simulink model "Model6"  (Simulink 8.1)
settings: Solver=ode15s  StartTime=StartTime  StopTime=StopTime  FixedStep=FixedStepSize  MaxStep=0.01  RelTol=1e-3
undefined symbols (not defined in the file or in its folder): D, dP, Ki, KOnline, Kp, M, R, TCH
settings Model: Creator=posq  LastModifiedBy=mfal  ExtModeAutoUpdateStatusClock=off
settings DataIOCC: SaveTime=off
settings OptimizationCC: ExpressionDepthLimit=128  InitFltsAndDblsToZero=on
settings DebuggingCC: SaveWithParameterizedLinksMsg=none  MultiTaskCondExecSysMsg=none  StrictBusMsg=Warning
settings RTWCC: IncludeERTFirstTime=on

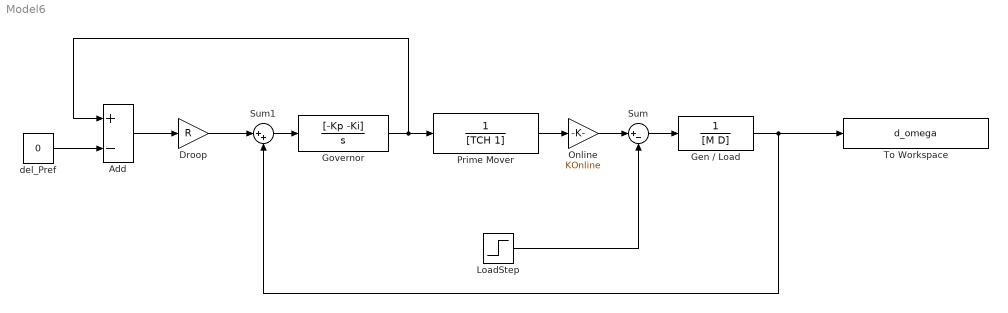
== system Model6 ==
  Add : Sum  Inputs=+-
  Droop : Gain  Gain=R
  Gen / Load : TransferFcn  Denominator=[M D]
  Governor : TransferFcn  Numerator=[-Kp -Ki]  Denominator=[1 0]
  LoadStep : Step  Time=0  After=dP  SampleTime=0
  Online : Gain  Gain=KOnline
  Prime Mover : TransferFcn  Denominator=[TCH 1]
  Sum : Sum  Inputs=|+-
  Sum1 : Sum  Inputs=|++
  To Workspace : ToWorkspace  VariableName=d_omega  SampleTime=-1  SaveFormat=Structure With Time
  del_Pref : Constant  Value=0
  wires:
  Gen / Load/1 -> To Workspace/1, Sum1/2
  Sum/1 -> Gen / Load/1
  LoadStep/1 -> Sum/2
  Governor/1 -> Prime Mover/1, Add/1
  Sum1/1 -> Governor/1
  Droop/1 -> Sum1/1
  Add/1 -> Droop/1
  del_Pref/1 -> Add/2
  Prime Mover/1 -> Online/1
  Online/1 -> Sum/1
